simulink model "System_Adjoint"  (R2016b)
settings: Solver=FixedStepAuto  StartTime=0.0  StopTime=tF  FixedStep=0.01  RelTol=1e-3
values from neighbouring files (symbols this model uses):
  dt = 1e-7    (= 1e-07)    [parameters.m]
  K = K_r(i)    [Proj_1a.m]    (also in Proj_1b.m; Proj_5.m = K_i(i))
  K_dth = 0.05    [Proj_1b.m]    (also in Proj_5.m = -0.04; parameters.m = 0.05*sgn)
  M_d = M_d_r(i)    [Proj_7.m]    (also in parameters.m = 200*sgn)
  N = 3    [parameters.m]
  rho_v = rho_i(i)    [Proj_2.m]    (also in Proj_2_3.m; Proj_3.m; Proj_5.m = 10; Proj_6.m = 10)
  rho_w = 10^-4    (= 0.0001)    [parameters.m]
  T_m = 120    [parameters.m]
  tau = tau_i(i)    [Proj_4.m]    (also in parameters.m = 0.05)
  Vc = 1250    [parameters.m]
settings Model: Creator=Daniel  LastModifiedBy=Daniel

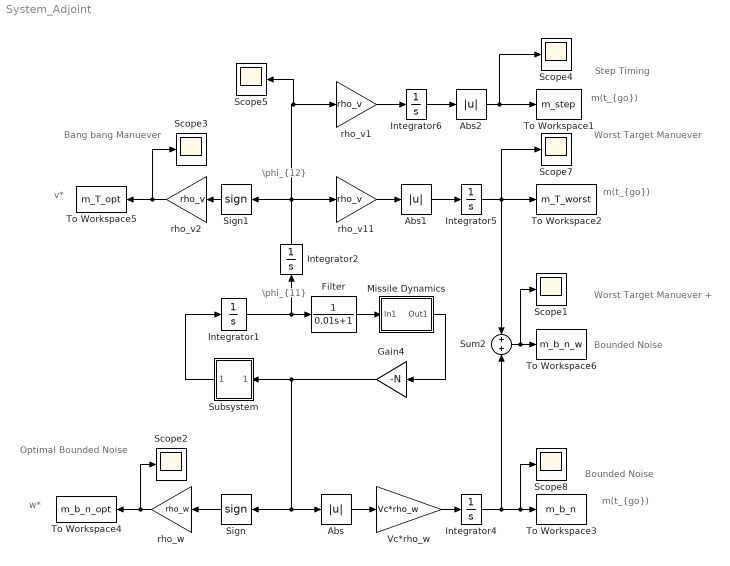
== system System_Adjoint ==
  note: Step Timing
  note: \phi_{11}
  note: Worst Target
      | Manuever
  note: Bounded Noise
  note: w*
  note: m(t_{go})
  note: m(t_{go})
  note: v*
  note: \phi_{12}
  note: m(t_{go})
  note: Bang bang
      | Manuever
  note: Optimal Bounded
      | Noise
  note: Worst Target
      | Manuever
      | +
  note: Bounded Noise
  Abs : Abs
  Abs1 : Abs
  Abs2 : Abs
  Filter : TransferFcn  Numerator=1  Denominator=[0.01 1]
  Gain4 : Gain  Gain=-N
  Integrator1 : Integrator  InitialCondition=1
  Integrator{2,4..6} (4 alike) : Integrator
  Missile Dynamics : Subsystem
      mask Display: image('Gm_s.PNG');
  Scope{1..5,7..8} (7 alike) : Scope
  Sign : Signum
  Sign1 : Signum
  Subsystem : Subsystem
      mask Display: image('t_go.PNG');
  Sum2 : Sum  Inputs=+|+
  To Workspace1 : ToWorkspace  VariableName=m_step  SaveFormat=Timeseries  SampleTime=-1
  To Workspace2 : ToWorkspace  VariableName=m_T_worst  SaveFormat=Timeseries  SampleTime=-1
  To Workspace3 : ToWorkspace  VariableName=m_b_n  SaveFormat=Timeseries  SampleTime=-1
  To Workspace4 : ToWorkspace  VariableName=m_b_n_opt  SaveFormat=Timeseries  SampleTime=-1
  To Workspace5 : ToWorkspace  VariableName=m_T_opt  SaveFormat=Timeseries  SampleTime=-1
  To Workspace6 : ToWorkspace  VariableName=m_b_n_w  SaveFormat=Timeseries  SampleTime=-1
  Vc*rho_w : Gain  Gain=Vc*rho_w
  rho_v1 : Gain  Gain=rho_v
  rho_v11 : Gain  Gain=rho_v
  rho_v2 : Gain  Gain=rho_v
  rho_w : Gain  Gain=rho_w
  wires:
  Subsystem/1(t_go) -> Integrator1/1
  Integrator2/1 -> Scope5/1, rho_v1/1, Sign1/1, rho_v11/1
  Gain4/1 -> Abs/1, Sign/1, Subsystem/1(In1)
  Abs/1 -> Vc*rho_w/1
  Vc*rho_w/1 -> Integrator4/1
  Integrator4/1 -> Sum2/2, Scope8/1, To Workspace3/1
  Sign/1 -> rho_w/1
  rho_w/1 -> Scope2/1, To Workspace4/1
  rho_v11/1 -> Abs1/1
  Abs1/1 -> Integrator5/1
  Integrator5/1 -> To Workspace2/1, Scope7/1, Sum2/1
  rho_v1/1 -> Integrator6/1
  Integrator6/1 -> Abs2/1
  Abs2/1 -> To Workspace1/1, Scope4/1
  Sign1/1 -> rho_v2/1
  rho_v2/1 -> To Workspace5/1, Scope3/1
  Integrator1/1 -> Filter/1, Integrator2/1
  Missile Dynamics/1(Out1) -> Gain4/1
  Sum2/1 -> To Workspace6/1, Scope1/1
  Filter/1 -> Missile Dynamics/1(In1)

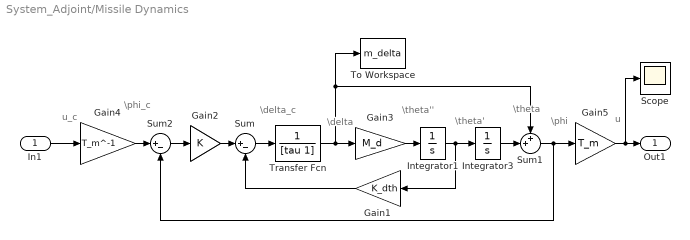
== system System_Adjoint/Missile Dynamics ==
  note: \theta'
  note: \theta''
  note: \theta
  note: \delta
  note: \delta_c
  note: \phi_c
  note: \phi
  note: u
  note: u_c
  In1 : Inport
  Gain1 : Gain  Gain=K_dth
  Gain2 : Gain  Gain=K
  Gain3 : Gain  Gain=M_d
  Gain4 : Gain  Gain=T_m^-1
  Gain5 : Gain  Gain=T_m
  Integrator1 : Integrator
  Integrator3 : Integrator
  Scope : Scope
  Sum : Sum  Inputs=|+-
  Sum1 : Sum  Inputs=++|
  Sum2 : Sum  Inputs=|+-
  To Workspace : ToWorkspace  VariableName=m_delta  SaveFormat=Timeseries  SampleTime=-1
  Transfer Fcn : TransferFcn  Denominator=[tau 1]
  Out1 : Outport
  wires:
  Gain1/1 -> Sum/2
  Sum/1 -> Transfer Fcn/1
  Gain2/1 -> Sum/1
  Transfer Fcn/1 -> Sum1/1, To Workspace/1, Gain3/1
  Sum1/1 -> Sum2/2, Gain5/1
  Gain3/1 -> Integrator1/1
  Integrator1/1 -> Integrator3/1, Gain1/1
  Integrator3/1 -> Sum1/2
  Sum2/1 -> Gain2/1
  Gain5/1 -> Scope/1, Out1/1
  In1/1 -> Gain4/1
  Gain4/1 -> Sum2/1

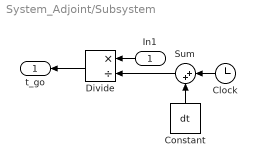
== system System_Adjoint/Subsystem ==
  In1 : Inport
  Clock : Clock
  Constant : Constant  Value=dt
  Divide : Product  Inputs=*/
  Sum : Sum  Inputs=|++
  t_go : Outport
  wires:
  Sum/1 -> Divide/2
  In1/1 -> Divide/1
  Divide/1 -> t_go/1
  Constant/1 -> Sum/2
  Clock/1 -> Sum/1
